simulink model "ARINC429_DW"  (R2020b)
settings: Solver=VariableStepAuto  StartTime=0.0  StopTime=10.0  RelTol=1e-3
(part 2 of 2)

== system ARINC429_DW/Encoder/Modulo10 /Subsystem ==
  In1 : Inport
  Data Type Conversion : DataTypeConversion  OutDataTypeStr=uint8
  Divide1 : Product  Inputs=*/
  Float Const2 : Constant  Value=10  OutDataTypeStr=single
  Product : Product
  Subtract : Sum  Inputs=+-
  Out1 : Outport
  Out2 : Outport  Port=2
  wires:
  Data Type Conversion/1 -> Out2/1, Subtract/2
  Float Const2/1 -> [F_10]
  Divide1/1 -> Subtract/1, Data Type Conversion/1
  Product/1 -> Out1/1
  Subtract/1 -> Product/1
  In1/1 -> Divide1/1
  [F_10] -> Divide1/2
  [F_10] -> Product/2

== system ARINC429_DW/Encoder/Modulo10 /Subsystem1 ==
  In1 : Inport
  Data Type Conversion1 : DataTypeConversion  OutDataTypeStr=uint8
  Divide2 : Product  Inputs=*/
  Float Const2 : Constant  Value=10  OutDataTypeStr=single
  Product1 : Product
  Subtract1 : Sum  Inputs=+-
  Out1 : Outport
  Out2 : Outport  Port=2
  wires:
  Float Const2/1 -> [F_10]
  Data Type Conversion1/1 -> Out2/1, Subtract1/2
  In1/1 -> Divide2/1
  [F_10] -> Divide2/2
  [F_10] -> Product1/2
  Divide2/1 -> Subtract1/1, Data Type Conversion1/1
  Subtract1/1 -> Product1/1
  Product1/1 -> Out1/1

== system ARINC429_DW/Encoder/Modulo10 /Subsystem2 ==
  In1 : Inport
  Data Type Conversion2 : DataTypeConversion  OutDataTypeStr=uint8
  Divide3 : Product  Inputs=*/
  Float Const1 : Constant  Value=10  OutDataTypeStr=single
  Product2 : Product
  Subtract2 : Sum  Inputs=+-
  Out1 : Outport
  wires:
  Product2/1 -> Out1/1
  [F_10] -> Product2/2
  In1/1 -> Divide3/1
  Data Type Conversion2/1 -> Subtract2/2
  Subtract2/1 -> Product2/1
  Divide3/1 -> Data Type Conversion2/1, Subtract2/1
  Float Const1/1 -> [F_10]
  [F_10] -> Divide3/2

== system ARINC429_DW/Encoder/base 8 encoder/Subsystem ==
  In1 : Inport
  Subsystem : Subsystem
  Subsystem1 : Subsystem
  Out1 : Outport
  Out2 : Outport  Port=2
  wires:
  In1/1 -> Subsystem/1(In1)
  Subsystem/1(Out1) -> Out1/1
  Subsystem/2(Out2) -> Subsystem1/1(In1)
  Subsystem1/1(Out1) -> Out2/1

== system ARINC429_DW/Encoder/base 8 encoder/Subsystem1 ==
  In1 : Inport
  Subsystem : Subsystem
  Subsystem1 : Subsystem
  Subsystem2 : Subsystem
  Out1 : Outport
  Out2 : Outport  Port=2
  Out3 : Outport  Port=3
  wires:
  In1/1 -> Subsystem/1(In1)
  Subsystem/1(Out1) -> Out1/1
  Subsystem/2(Out2) -> Subsystem1/1(In1)
  Subsystem1/1(Out1) -> Out2/1
  Subsystem1/2(Out2) -> Subsystem2/1(In1)
  Subsystem2/1(Out1) -> Out3/1

== system ARINC429_DW/Encoder/base 8 encoder/Subsystem2 ==
  In1 : Inport
  Subsystem : Subsystem
  Subsystem1 : Subsystem
  Subsystem2 : Subsystem
  Out1 : Outport
  Out2 : Outport  Port=2
  Out3 : Outport  Port=3
  wires:
  In1/1 -> Subsystem/1(In1)
  Subsystem/1(Out1) -> Out1/1
  Subsystem/2(Out2) -> Subsystem1/1(In1)
  Subsystem1/1(Out1) -> Out2/1
  Subsystem1/2(Out2) -> Subsystem2/1(In1)
  Subsystem2/1(Out1) -> Out3/1

== system ARINC429_DW/Encoder/base 8 encoder/Subsystem/Subsystem ==
  In1 : Inport
  Data Type Conversion : DataTypeConversion  OutDataTypeStr=uint8
  Data Type Conversion15 : DataTypeConversion  OutDataTypeStr=uint8
  Divide1 : Product  Inputs=*/
  Divide2 : Product  Inputs=*/
  Float Const : Constant  Value=2  OutDataTypeStr=single
  Float Const1 : Constant  Value=0.5  OutDataTypeStr=single
  Subtract : Sum  Inputs=+-
  Out1 : Outport
  Out2 : Outport  Port=2
  wires:
  Data Type Conversion/1 -> Out2/1, Subtract/2
  Data Type Conversion15/1 -> Out1/1
  Float Const1/1 -> Divide2/2
  [F_2] -> Divide1/2
  Float Const/1 -> [F_2]
  Divide1/1 -> Subtract/1, Data Type Conversion/1
  In1/1 -> Divide1/1
  Subtract/1 -> Divide2/1
  Divide2/1 -> Data Type Conversion15/1

== system ARINC429_DW/Encoder/base 8 encoder/Subsystem/Subsystem1 ==
  In1 : Inport
  Data Type Conversion1 : DataTypeConversion  OutDataTypeStr=uint8
  Data Type Conversion14 : DataTypeConversion  OutDataTypeStr=uint8
  Divide3 : Product  Inputs=*/
  Divide4 : Product  Inputs=*/
  Float Const : Constant  Value=1.99  OutDataTypeStr=single
  Float Const2 : Constant  Value=0.5  OutDataTypeStr=single
  Subtract2 : Sum  Inputs=+-
  Out1 : Outport
  wires:
  Divide3/1 -> Subtract2/1, Data Type Conversion1/1
  Data Type Conversion14/1 -> Out1/1
  [F_2] -> Divide3/2
  Divide4/1 -> Data Type Conversion14/1
  Subtract2/1 -> Divide4/1
  Float Const2/1 -> Divide4/2
  Data Type Conversion1/1 -> Subtract2/2
  In1/1 -> Divide3/1
  Float Const/1 -> [F_2]

== system ARINC429_DW/Encoder/base 8 encoder/Subsystem1/Subsystem ==
  In1 : Inport
  Data Type Conversion2 : DataTypeConversion  OutDataTypeStr=uint8
  Data Type Conversion8 : DataTypeConversion  OutDataTypeStr=uint8
  Divide5 : Product  Inputs=*/
  Divide6 : Product  Inputs=*/
  Float Const : Constant  Value=1.99  OutDataTypeStr=single
  Float Const3 : Constant  Value=0.4999  OutDataTypeStr=single
  Subtract1 : Sum  Inputs=+-
  Out1 : Outport
  Out2 : Outport  Port=2
  wires:
  Divide5/1 -> Data Type Conversion2/1, Subtract1/1
  Float Const/1 -> [F_2]
  Divide6/1 -> Data Type Conversion8/1
  Data Type Conversion8/1 -> Out1/1
  Float Const3/1 -> Divide6/2
  Data Type Conversion2/1 -> Out2/1, Subtract1/2
  Subtract1/1 -> Divide6/1
  In1/1 -> Divide5/1
  [F_2] -> Divide5/2

== system ARINC429_DW/Encoder/base 8 encoder/Subsystem1/Subsystem1 ==
  In1 : Inport
  Data Type Conversion13 : DataTypeConversion  OutDataTypeStr=uint8
  Data Type Conversion3 : DataTypeConversion  OutDataTypeStr=uint8
  Divide7 : Product  Inputs=*/
  Divide8 : Product  Inputs=*/
  Float Const : Constant  Value=1.99  OutDataTypeStr=single
  Float Const4 : Constant  Value=0.5  OutDataTypeStr=single
  Subtract3 : Sum  Inputs=+-
  Out1 : Outport
  Out2 : Outport  Port=2
  wires:
  Divide8/1 -> Data Type Conversion13/1
  Float Const4/1 -> Divide8/2
  Divide7/1 -> Subtract3/1, Data Type Conversion3/1
  [F_2] -> Divide7/2
  Subtract3/1 -> Divide8/1
  Data Type Conversion3/1 -> Out2/1, Subtract3/2
  In1/1 -> Divide7/1
  Data Type Conversion13/1 -> Out1/1
  Float Const/1 -> [F_2]

== system ARINC429_DW/Encoder/base 8 encoder/Subsystem1/Subsystem2 ==
  In1 : Inport
  Data Type Conversion12 : DataTypeConversion  OutDataTypeStr=uint8
  Data Type Conversion4 : DataTypeConversion  OutDataTypeStr=uint8
  Divide10 : Product  Inputs=*/
  Divide9 : Product  Inputs=*/
  Float Const : Constant  Value=1.99  OutDataTypeStr=single
  Float Const5 : Constant  Value=0.5  OutDataTypeStr=single
  Subtract4 : Sum  Inputs=+-
  Out1 : Outport
  wires:
  In1/1 -> Divide9/1
  Subtract4/1 -> Divide10/1
  Divide9/1 -> Subtract4/1, Data Type Conversion4/1
  Divide10/1 -> Data Type Conversion12/1
  Float Const5/1 -> Divide10/2
  [F_2] -> Divide9/2
  Data Type Conversion12/1 -> Out1/1
  Float Const/1 -> [F_2]
  Data Type Conversion4/1 -> Subtract4/2

== system ARINC429_DW/Encoder/base 8 encoder/Subsystem2/Subsystem ==
  In1 : Inport
  Data Type Conversion5 : DataTypeConversion  OutDataTypeStr=uint8
  Data Type Conversion9 : DataTypeConversion  OutDataTypeStr=uint8
  Divide12 : Product  Inputs=*/
  Divide13 : Product  Inputs=*/
  Float Const : Constant  Value=1.99  OutDataTypeStr=single
  Float Const6 : Constant  Value=0.50  OutDataTypeStr=single
  Subtract5 : Sum  Inputs=+-
  Out1 : Outport
  Out2 : Outport  Port=2
  wires:
  Divide12/1 -> Subtract5/1, Data Type Conversion5/1
  [F_2] -> Divide12/2
  Data Type Conversion9/1 -> Out1/1
  Data Type Conversion5/1 -> Out2/1, Subtract5/2
  Subtract5/1 -> Divide13/1
  Divide13/1 -> Data Type Conversion9/1
  In1/1 -> Divide12/1
  Float Const/1 -> [F_2]
  Float Const6/1 -> Divide13/2

== system ARINC429_DW/Encoder/base 8 encoder/Subsystem2/Subsystem1 ==
  In1 : Inport
  Data Type Conversion10 : DataTypeConversion  OutDataTypeStr=uint8
  Data Type Conversion6 : DataTypeConversion  OutDataTypeStr=uint8
  Divide14 : Product  Inputs=*/
  Divide15 : Product  Inputs=*/
  Float Const : Constant  Value=1.99  OutDataTypeStr=single
  Float Const7 : Constant  Value=0.5  OutDataTypeStr=single
  Subtract6 : Sum  Inputs=+-
  Out1 : Outport
  Out2 : Outport  Port=2
  wires:
  Subtract6/1 -> Divide15/1
  Data Type Conversion6/1 -> Subtract6/2, Out2/1
  Float Const7/1 -> Divide15/2
  Divide14/1 -> Subtract6/1, Data Type Conversion6/1
  Divide15/1 -> Data Type Conversion10/1
  [F_2] -> Divide14/2
  In1/1 -> Divide14/1
  Data Type Conversion10/1 -> Out1/1
  Float Const/1 -> [F_2]

== system ARINC429_DW/Encoder/base 8 encoder/Subsystem2/Subsystem2 ==
  In1 : Inport
  Data Type Conversion11 : DataTypeConversion  OutDataTypeStr=uint8
  Data Type Conversion7 : DataTypeConversion  OutDataTypeStr=uint8
  Divide11 : Product  Inputs=*/
  Divide16 : Product  Inputs=*/
  Float Const : Constant  Value=1.99  OutDataTypeStr=single
  Float Const8 : Constant  Value=0.49  OutDataTypeStr=single
  Subtract7 : Sum  Inputs=+-
  Out1 : Outport
  wires:
  Divide11/1 -> Data Type Conversion11/1
  Divide16/1 -> Subtract7/1, Data Type Conversion7/1
  Subtract7/1 -> Divide11/1
  [F_2] -> Divide16/2
  Float Const/1 -> [F_2]
  In1/1 -> Divide16/1
  Data Type Conversion7/1 -> Subtract7/2
  Float Const8/1 -> Divide11/2
  Data Type Conversion11/1 -> Out1/1
